simulink model "cvoo_g19_controlo_altitude"  (R2020a)
settings: Solver=VariableStepAuto  StartTime=0.0  StopTime=10  RelTol=1e-3
values from neighbouring files (symbols this model uses):
  a = [ ... (first row only)    [main.m]    (also in main_gaspar.m; main_ze_rp1.m)
  b_sf = [ ... (first row only)    [main.m]    (also in main_gaspar.m)
  c = eye(size(a))    [main.m]    (also in main_gaspar.m; main_ze_rp1.m)
  d_sf = zeros(size(b_sf))    [main.m]    (also in main_gaspar.m)
  h_ref = fscanf(fileID,'    [ground_model.m]
  K_lqr = lqr(a_h_pt_int, b_h_pt_int, Q, R)    [main.m]    (also in main_gaspar.m = lqr(a_h_int, b_h_sf_int, Q, R))
  u_ref = 2    [main.m]    (also in main_gaspar.m = -5)
  x0 = [0 0 0 0]    [main.m]    (also in main_gaspar.m)
undefined symbols (not defined in the file or in its folder): cond_ini, max_deflec
settings Model: Creator=josem  LastModifiedBy=josem

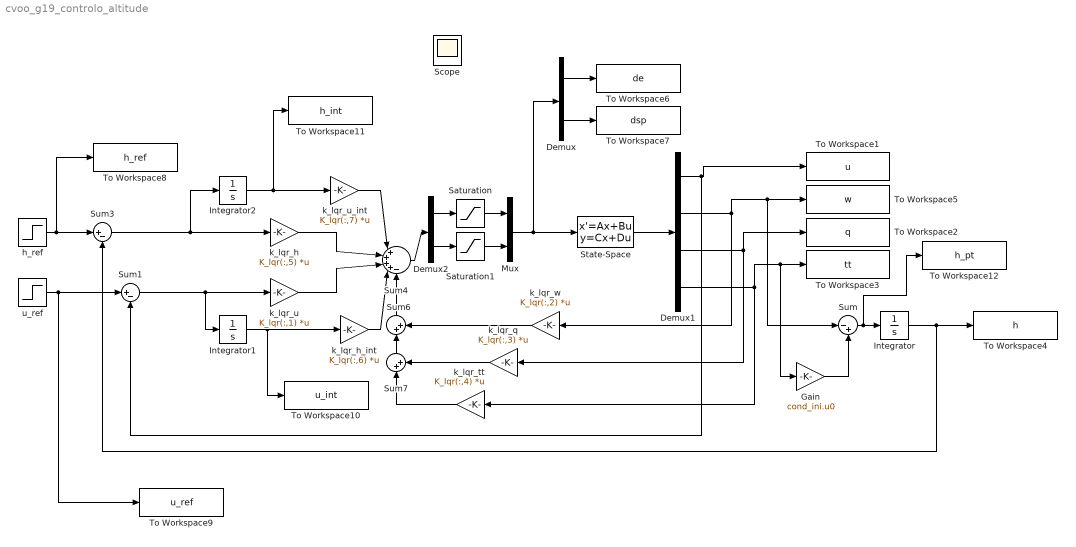
== system cvoo_g19_controlo_altitude ==
  Demux : Demux  Outputs=2
  Demux1 : Demux
  Demux2 : Demux  Outputs=2
  Gain : Gain  Gain=cond_ini.u0
  Integrator : Integrator
  Integrator1 : Integrator  UpperSaturationLimit=10  LowerSaturationLimit=-10
  Integrator2 : Integrator  UpperSaturationLimit=10  LowerSaturationLimit=-10
  Mux : Mux  Inputs=2
  Saturation : Saturate  UpperLimit=max_deflec.demax  LowerLimit=max_deflec.demin
  Saturation1 : Saturate  UpperLimit=max_deflec.spmax  LowerLimit=0
  State-Space : StateSpace  A=a  B=b_sf  C=c  D=d_sf  InitialCondition=x0
  Sum : Sum  Inputs=|-+
  Sum1 : Sum  Inputs=|+-
  Sum3 : Sum  Inputs=|+-
  Sum4 : Sum  Inputs=|++++-
  Sum6 : Sum  Inputs=|++
  Sum7 : Sum  Inputs=|++
  To Workspace1 : ToWorkspace  VariableName=u  SampleTime=-1
  To Workspace10 : ToWorkspace  VariableName=u_int  SampleTime=-1
  To Workspace11 : ToWorkspace  VariableName=h_int  SampleTime=-1
  To Workspace12 : ToWorkspace  VariableName=h_pt  SampleTime=-1
  To Workspace2 : ToWorkspace  VariableName=q  SampleTime=-1
  To Workspace3 : ToWorkspace  VariableName=tt  SampleTime=-1
  To Workspace4 : ToWorkspace  VariableName=h  SampleTime=-1
  To Workspace5 : ToWorkspace  VariableName=w  SampleTime=-1
  To Workspace6 : ToWorkspace  VariableName=de  SampleTime=-1
  To Workspace7 : ToWorkspace  VariableName=dsp  SampleTime=-1
  To Workspace8 : ToWorkspace  VariableName=h_ref  SampleTime=-1
  To Workspace9 : ToWorkspace  VariableName=u_ref  SampleTime=-1
  h_ref : Step  After=h_ref  SampleTime=0  VectorParams1D=off
  k_lqr_h : Gain  Gain=K_lqr(:,5)  Multiplication=Matrix(K*u)
  k_lqr_h_int : Gain  Gain=K_lqr(:,6)  Multiplication=Matrix(K*u)
  k_lqr_q : Gain  Gain=K_lqr(:,3)  Multiplication=Matrix(K*u)
  k_lqr_tt : Gain  Gain=K_lqr(:,4)  Multiplication=Matrix(K*u)
  k_lqr_u : Gain  Gain=K_lqr(:,1)  Multiplication=Matrix(K*u)
  k_lqr_u_int : Gain  Gain=K_lqr(:,7)  Multiplication=Matrix(K*u)
  k_lqr_w : Gain  Gain=K_lqr(:,2)  Multiplication=Matrix(K*u)
  u_ref : Step  Time=20  After=u_ref  SampleTime=0  VectorParams1D=off
  Scope : Scope
  wires:
  State-Space/1 -> Demux1/1
  Demux1/2 -> Sum/1, To Workspace5/1, k_lqr_w/1
  Demux1/3 -> k_lqr_q/1, To Workspace2/1
  Demux1/4 -> Gain/1, To Workspace3/1, k_lqr_tt/1
  h_ref/1 -> Sum3/1, To Workspace8/1
  k_lqr_h/1 -> Sum4/2
  k_lqr_w/1 -> Sum6/2
  Sum7/1 -> Sum6/1
  k_lqr_q/1 -> Sum7/2
  Sum6/1 -> Sum4/5
  Demux/1 -> To Workspace6/1
  Demux/2 -> To Workspace7/1
  Saturation1/1 -> Mux/2
  Demux2/2 -> Saturation1/1
  Demux2/1 -> Saturation/1
  Saturation/1 -> Mux/1
  Mux/1 -> Demux/1, State-Space/1
  Sum4/1 -> Demux2/1
  Gain/1 -> Sum/2
  Sum/1 -> To Workspace12/1, Integrator/1
  Integrator/1 -> Sum3/2, To Workspace4/1
  u_ref/1 -> To Workspace9/1, Sum1/1
  Demux1/1 -> Sum1/2, To Workspace1/1
  Integrator2/1 -> To Workspace11/1, k_lqr_u_int/1
  k_lqr_tt/1 -> Sum7/1
  Integrator1/1 -> To Workspace10/1, k_lqr_h_int/1
  k_lqr_u/1 -> Sum4/3
  k_lqr_h_int/1 -> Sum4/4
  k_lqr_u_int/1 -> Sum4/1
  Sum3/1 -> Integrator2/1, k_lqr_h/1
  Sum1/1 -> k_lqr_u/1, Integrator1/1
